simulink model "nuri3s_basic_model"  (R2024b)
settings: Solver=VariableStepAuto  StartTime=0.0  StopTime=10.0  RelTol=1e-3
libraries: robotmaniplib x1
settings Model: Creator=변재형  LastModifiedBy=변재형

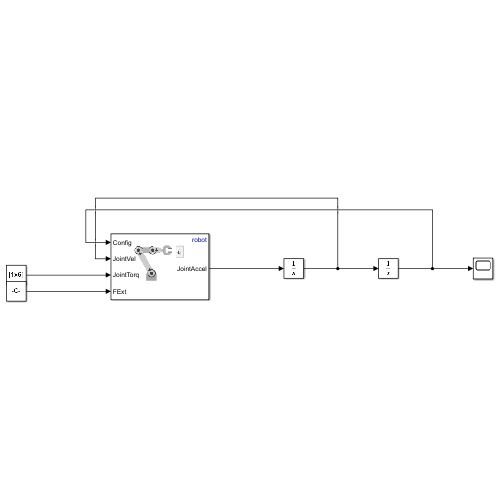
[thumbnail: Simulink's stored preview of the top-level diagram]
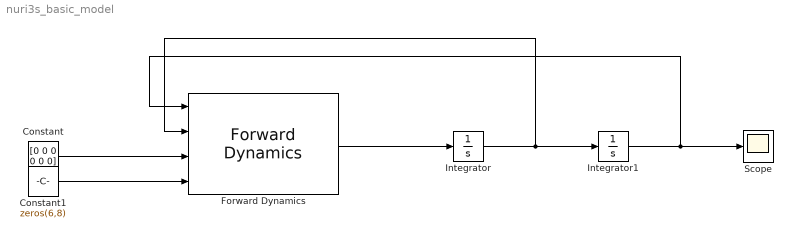
== system nuri3s_basic_model ==
  Constant : Constant  Value=[0 0 0 0 0 0]
  Constant1 : Constant  Value=zeros(6,8)
  Forward Dynamics : robotmaniplib/Forward Dynamics  RigidBodyTree=robot  SimulateUsing=Interpreted execution
  Integrator : Integrator
  Integrator1 : Integrator
  Scope : Scope
  wires:
  Forward Dynamics/1 -> Integrator/1
  Integrator/1 -> Forward Dynamics/2, Integrator1/1
  Integrator1/1 -> Forward Dynamics/1, Scope/1
  Constant/1 -> Forward Dynamics/3
  Constant1/1 -> Forward Dynamics/4
